simulink model "a6_4_solving_multiple_variable_equations"  (R2018a)
settings: Solver=VariableStepAuto  StartTime=0.0  StopTime=10.0  RelTol=1e-3
settings Model: Creator=r0x6f736f646f  LastModifiedBy=r0x6f736f646f

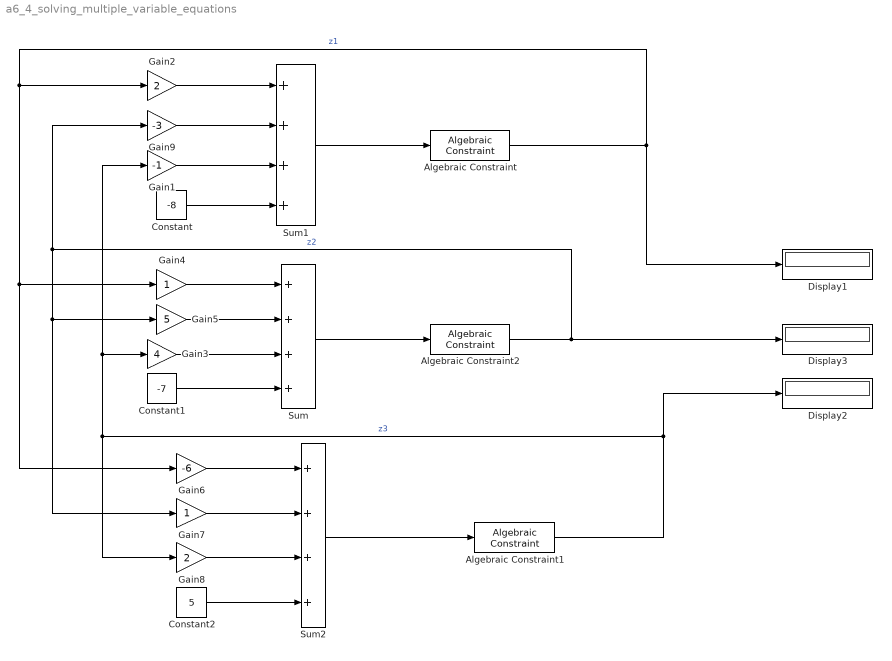
== system a6_4_solving_multiple_variable_equations ==
  Algebraic Constraint : AlgebraicConstraint
  Algebraic Constraint1 : AlgebraicConstraint
  Algebraic Constraint2 : AlgebraicConstraint
  Constant : Constant  Value=-8
  Constant1 : Constant  Value=-7
  Constant2 : Constant  Value=5
  Display1 : Display
  Display2 : Display
  Display3 : Display
  Gain1 : Gain  Gain=-1
  Gain2 : Gain  Gain=2
  Gain3 : Gain  Gain=4
  Gain4 : Gain
  Gain5 : Gain  Gain=5
  Gain6 : Gain  Gain=-6
  Gain7 : Gain
  Gain8 : Gain  Gain=2
  Gain9 : Gain  Gain=-3
  Sum : Sum  Inputs=++++
  Sum1 : Sum  Inputs=++++
  Sum2 : Sum  Inputs=++++
  wires:
  Sum1/1 -> Algebraic Constraint/1
  Sum2/1 -> Algebraic Constraint1/1
  Algebraic Constraint1/1 -> Gain3/1, Gain1/1, Gain8/1, Display2/1  "z3"
  Sum/1 -> Algebraic Constraint2/1
  Algebraic Constraint2/1 -> Gain9/1, Gain5/1, Gain7/1, Display3/1  "z2"
  Gain1/1 -> Sum1/3
  Gain2/1 -> Sum1/1
  Gain9/1 -> Sum1/2
  Gain3/1 -> Sum/3
  Gain5/1 -> Sum/2
  Gain4/1 -> Sum/1
  Gain6/1 -> Sum2/1
  Gain7/1 -> Sum2/2
  Gain8/1 -> Sum2/3
  Constant/1 -> Sum1/4
  Constant1/1 -> Sum/4
  Constant2/1 -> Sum2/4
  Algebraic Constraint/1 -> Display1/1, Gain2/1, Gain4/1, Gain6/1  "z1"
